simulink model "VSI_GT_avg_il_pll_sv"  (R2016a)
settings: Solver=ode23t  StartTime=0.0  StopTime=0.3  MaxStep=10e-6  RelTol=1e-4  AbsTol=1e-5
values from neighbouring files (symbols this model uses):
  Gdel = Gsvm    [ZVSI_il_tf_cal_sim_comp_frd_PLL_equation.m]    (also in ZVSI_il_tf_cal_sim_comp_frd_model_PQC.m; ZVSI_il_tf_cal_sim_comp_frd_model_v1.m; ZVSI_il_tf_pll_for_shuo.m; ZVSI_ol_pll_share.m)
  Id_ref = (P*Vsd_s-Q*Vsq_s)/(Vsd_s^2+Vsq_s^2)    [ZDQ_GT_DC.m]    (also in ZVSI_il_tf_cal_sim_comp_frd_PLL_equation.m = -10.04; ZVSI_il_tf_cal_sim_comp_frd_model_PQC.m; ZVSI_il_tf_cal_sim_comp_frd_model_v1.m = 1*Id_ref_a(2); ZVSI_il_tf_pll_for_shuo.m = -11.03)
  Iq_ref = (P*Vsq_s+Q*Vsd_s)/(Vsd_s^2+Vsq_s^2)    [ZDQ_GT_DC.m]    (also in ZVSI_il_tf_cal_sim_comp_frd_PLL_equation.m = 0; ZVSI_il_tf_cal_sim_comp_frd_model_PQC.m; ZVSI_il_tf_cal_sim_comp_frd_model_v1.m = 1*Iq_ref_a(2); ZVSI_il_tf_pll_for_shuo.m = 0)
  Ki = tf_filter_dq    [ZVSI_il_tf_cal_sim_comp_frd_PLL_equation.m]    (also in ZVSI_il_tf_cal_sim_comp_frd_model_PQC.m; ZVSI_il_tf_cal_sim_comp_frd_model_v1.m; ZVSI_il_tf_pll_for_shuo.m; ZVSI_ol_pll_zero_pole.m)
  kii = 2*pi*fi*RLboost_con/Vdcref    (= 5.11963247252)    [ZVSI_il_tf_cal_sim_comp_frd_PLL_equation.m]    (also in ZVSI_il_tf_cal_sim_comp_frd_model_PQC.m = ki_i(2)*2*pi*fi*RLboost_con/Vdcref; ZVSI_il_tf_cal_sim_comp_frd_model_v1.m = ki_i(2)*2*pi*fi*RLboost_con/Vdcref; ZVSI_il_tf_pll_for_shuo.m = 25.5982)
  kpi = 2*pi*fi*Lboost_con/Vdcref    (= 0.0465421133865)    [ZVSI_il_tf_cal_sim_comp_frd_PLL_equation.m]    (also in ZVSI_il_tf_cal_sim_comp_frd_model_PQC.m = 0.0232710566933; ZVSI_il_tf_cal_sim_comp_frd_model_v1.m = 0.0232710566933; ZVSI_il_tf_pll_for_shuo.m = 0.0233)
  Kv = tf_filter_dq    [ZVSI_il_tf_cal_sim_comp_frd_PLL_equation.m]    (also in ZVSI_il_tf_cal_sim_comp_frd_model_PQC.m; ZVSI_il_tf_cal_sim_comp_frd_model_v1.m; ZVSI_il_tf_pll_for_shuo.m; ZVSI_ol_pll_zero_pole.m)
  L = 1000e-6    (= 0.001)    [LC_parallel.m]    (also in ZVSI_il_tf_cal_sim_comp_frd_PLL_equation.m; ZVSI_il_tf_cal_sim_comp_frd_model_PQC.m = 0.00097; ZVSI_il_tf_cal_sim_comp_frd_model_v1.m; ZVSI_il_tf_pll_for_shuo.m)
  Lboost_con = 1000e-6    (= 0.001)    [ZVSI_il_tf_cal_sim_comp_frd_PLL_equation.m]    (also in ZVSI_il_tf_cal_sim_comp_frd_model_PQC.m; ZVSI_il_tf_cal_sim_comp_frd_model_v1.m; ZVSI_il_tf_pll_for_shuo.m)
  omega = 2*pi*f    (= 376.991118431)    [ZVSI_il_tf_cal_sim_comp_frd_PLL_equation.m]    (also in ZVSI_il_tf_cal_sim_comp_frd_model_PQC.m = 2513.27412287; ZVSI_il_tf_cal_sim_comp_frd_model_v1.m = 2513.27412287; ZVSI_il_tf_pll_for_shuo.m = 2513.27412287; ZVSI_ol_pll_share.m = 2513.27412287)
  RL = 110e-3    (= 0.11)    [ZVSI_il_tf_cal_sim_comp_frd_PLL_equation.m]    (also in ZVSI_il_tf_cal_sim_comp_frd_model_PQC.m = 0.12; ZVSI_il_tf_cal_sim_comp_frd_model_v1.m; ZVSI_il_tf_pll_for_shuo.m; ZVSI_ol_pll_share.m)
  Vdcref = 270    [ZVSI_il_tf_cal_sim_comp_frd_PLL_equation.m]    (also in ZVSI_il_tf_cal_sim_comp_frd_model_PQC.m; ZVSI_il_tf_cal_sim_comp_frd_model_v1.m; ZVSI_il_tf_pll_for_shuo.m; ZVSI_ol_pll_share.m)
  Vsd_s = Vsdq(1)    [ZDQ_GT_DC.m]    (also in ZVSI_il_tf_cal_sim_comp_frd_PLL_equation.m; ZVSI_il_tf_cal_sim_comp_frd_model_PQC.m; ZVSI_il_tf_cal_sim_comp_frd_model_v1.m; ZVSI_il_tf_pll_for_shuo.m)
libraries: powerlib x23, cstblocks x13, simulink x3
settings Model: Creator=marko  LastModifiedBy=mchssbw3
settings SolverCC: ZeroCrossAlgorithm=Adaptive
settings DataIOCC: LimitDataPoints=on  SaveFormat=Array  SignalLoggingSaveFormat=ModelDataLogs
settings OptimizationCC: BlockReduction=off  DefaultParameterBehavior=Inlined  BufferReuse=off  ExpressionDepthLimit=2147483647
settings DebuggingCC: AlgebraicLoopMsg=none  UnderspecifiedInitializationDetection=Classic  MergeDetectMultiDrivingBlocksExec=none  MultiTaskDSMMsg=warning  MultiTaskCondExecSysMsg=none  UnconnectedInputMsg=none  UnconnectedOutputMsg=none  UnconnectedLineMsg=none  StateNameClashWarn=warning
settings HardwareCC: ProdBitPerPointer=32  ProdLargestAtomicFloat=None  ProdIntDivRoundTo=Undefined  ProdEndianess=Unspecified  ProdWordSize=32  ProdHWDeviceType=32-bit Generic
settings ModelReferenceCC: PropagateSignalLabelsOutOfModel=off
settings GRTTargetCC: CombineOutputUpdateFcns=off  GRTInterface=on
settings ConfigComp: CovModelRefEnable=Off

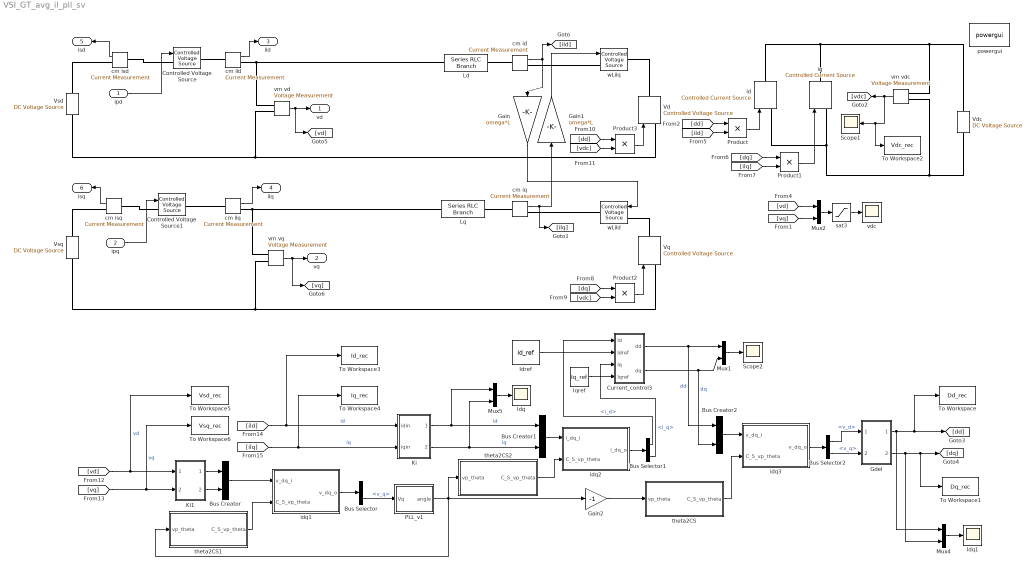
== system VSI_GT_avg_il_pll_sv ==
  ipd : Inport
  ipq : Inport  Port=2
  Bus Creator : BusCreator  Inputs=2
  Bus Creator1 : BusCreator  Inputs=2
  Bus Creator2 : BusCreator  Inputs=2
  Bus Selector : BusSelector  OutputSignals=v_d,v_q
  Bus Selector1 : BusSelector  OutputSignals=i_d,i_q
  Bus Selector2 : BusSelector  OutputSignals=v_d,v_q
  Controlled Voltage Source : powerlib/Electrical Sources/Controlled Voltage Source  Initialize=on  Source_Type=AC  Amplitude=0  Phase=0  Frequency=0  Measurements=None
  Controlled Voltage Source1 : powerlib/Electrical Sources/Controlled Voltage Source  Initialize=on  Source_Type=AC  Amplitude=0  Phase=0  Frequency=0  Measurements=None
  Current_control3 : Subsystem
  Gain : Gain  Gain=omega*L
  Gain1 : Gain  Gain=omega*L
  Gain2 : Gain  Gain=-1
  Gdel : Subsystem
  Idq : Scope
  Idq1 : Scope
  Idref : Constant  Value=Id_ref
  Iqref : Constant  Value=Iq_ref
  Ki : Subsystem
  Ki1 : Subsystem
  Ld : powerlib/Elements/Series RLC Branch  LConnTagsString=__new0  RConnTagsString=__new0  BranchType=RL  Resistance=RL  Inductance=L  SetiL0=off  InitialCurrent=0  Capacitance=1e-6  Setx0=off  InitialVoltage=0  Measurements=None
  Lq : powerlib/Elements/Series RLC Branch  LConnTagsString=__new0  RConnTagsString=__new0  BranchType=RL  Resistance=RL  Inductance=L  SetiL0=off  InitialCurrent=0  Capacitance=1e-6  Setx0=off  InitialVoltage=0  Measurements=None
  Mux{1..2,4..5} (4 alike) : Mux  Inputs=2
  PLL_v1 : Subsystem
  Product{,1..3} (4 alike) : Product  RndMeth=Zero
  Scope1 : Scope
  Scope2 : Scope
  To Workspace : ToWorkspace  VariableName=Dd_rec  SampleTime=-1
  To Workspace1 : ToWorkspace  VariableName=Dq_rec  SampleTime=-1
  To Workspace2 : ToWorkspace  VariableName=Vdc_rec  SampleTime=-1
  To Workspace3 : ToWorkspace  VariableName=Id_rec  SampleTime=-1
  To Workspace4 : ToWorkspace  VariableName=Iq_rec  SampleTime=-1
  To Workspace5 : ToWorkspace  VariableName=Vsd_rec  SampleTime=-1
  To Workspace6 : ToWorkspace  VariableName=Vsq_rec  SampleTime=-1
  Vd : powerlib/Electrical Sources/Controlled Voltage Source  Initialize=on  Source_Type=DC  Amplitude=0  Phase=0  Frequency=0  Measurements=None
  Vdc : powerlib/Electrical Sources/DC Voltage Source  Amplitude=270  Measurements=None
  Vq : powerlib/Electrical Sources/Controlled Voltage Source  Initialize=on  Source_Type=DC  Amplitude=0  Phase=0  Frequency=0  Measurements=None
  Vsd : powerlib/Electrical Sources/DC Voltage Source  Amplitude=Vsd_s  Measurements=None
  Vsq : powerlib/Electrical Sources/DC Voltage Source  Amplitude=0  Measurements=None
  cm id : powerlib/Measurements/Current Measurement  PhasorSimulation=off  OutputType=Complex  PSBequivalent=0
  cm ild : powerlib/Measurements/Current Measurement  PhasorSimulation=off  OutputType=Complex  PSBequivalent=0
  cm ilq : powerlib/Measurements/Current Measurement  PhasorSimulation=off  OutputType=Complex  PSBequivalent=0
  cm iq : powerlib/Measurements/Current Measurement  PhasorSimulation=off  OutputType=Complex  PSBequivalent=0
  cm isd : powerlib/Measurements/Current Measurement  PhasorSimulation=off  OutputType=Complex  PSBequivalent=0
  cm isq : powerlib/Measurements/Current Measurement  PhasorSimulation=off  OutputType=Complex  PSBequivalent=0
  id : powerlib/Electrical Sources/Controlled Current Source  Initialize=on  Source_Type=DC  Amplitude=0  Phase=0  Frequency=0  Measurements=None
  idq1 : Subsystem
  idq2 : Subsystem
  idq3 : Subsystem
  iq : powerlib/Electrical Sources/Controlled Current Source  Initialize=on  Source_Type=DC  Amplitude=0  Phase=0  Frequency=0  Measurements=None
  powergui : powerlib/powergui  Priority=1  SimulationMode=Continuous  SolverType=Tustin  SampleTime=50e-6  frequency=60  SPID=off  DisableSnubberDevices=off  DisableRonSwitches=off  DisableVfSwitches=off  SwTol=0  DisplayEquations=off  Interpol=off  ExternalGateDelay=off  methode=off  Ts=0  FunctionMessages=off  echomessages=off  HookPort=off  EnableUseOfTLC=off  x0status=blocks  frequencyindice=0  Pbase=100e6  ErrMax=1e-4  Iterations=50  UnitsV=kV  UnitsW=MW  buscounter=0  RestoreLinks=warning  ResistiveCurrentMeasurement=off  Frange=[0:2:500]  Ylog=off  Xlog=on  ShowGrid=off  save=off  variable=ZData  structure=0  ZoomFFT=on  StartTime=0.0  cycles=1  DisplayStyle=1  fundamental=60  FreqAxis=off  MaxFrequency=1000  frequencyindicesteady=1  RmsSteady=1  display=off
  sat3 : Saturate  UpperLimit=1000  LowerLimit=0
  theta2CS : Subsystem
  theta2CS1 : Subsystem
  theta2CS2 : Subsystem
  vdc : Scope
  vm vd : powerlib/Measurements/Voltage Measurement  PhasorSimulation=off  OutputType=Complex  PSBequivalent=0
  vm vdc : powerlib/Measurements/Voltage Measurement  PhasorSimulation=off  OutputType=Complex  PSBequivalent=0
  vm vq : powerlib/Measurements/Voltage Measurement  PhasorSimulation=off  OutputType=Complex  PSBequivalent=0
  wLild : powerlib/Electrical Sources/Controlled Voltage Source  Initialize=on  Source_Type=DC  Amplitude=0  Phase=0  Frequency=0  Measurements=None
  wLilq : powerlib/Electrical Sources/Controlled Voltage Source  Initialize=on  Source_Type=DC  Amplitude=0  Phase=0  Frequency=0  Measurements=None
  vd : Outport
  vq : Outport  Port=2
  ild : Outport  Port=3
  ilq : Outport  Port=4
  isd : Outport  Port=5
  isq : Outport  Port=6
  wires:
  cm id/1 -> Gain/1, [ild]
  Gain1/1 -> wLilq/1
  cm iq/1 -> [ilq], Gain1/1
  Gain/1 -> wLild/1
  vm vdc/1 -> [vdc], Scope1/1, To Workspace2/1
  Product/1 -> id/1
  [dd] -> Product/1
  [ild] -> Product/2
  Product1/1 -> iq/1
  [dq] -> Product1/1
  [ilq] -> Product1/2
  [dq] -> Product2/1
  [vdc] -> Product2/2
  Product2/1 -> Vq/1
  [dd] -> Product3/1
  [vdc] -> Product3/2
  Product3/1 -> Vd/1
  vm vd/1 -> vd/1, [vd]
  vm vq/1 -> vq/1, [vq]
  cm ild/1 -> ild/1
  cm ilq/1 -> ilq/1
  cm isd/1 -> isd/1
  cm isq/1 -> isq/1
  Current_control3/1(dd) -> Mux1/1, Bus Creator2/1  "dd"
  Current_control3/2(dq) -> Mux1/2, Bus Creator2/2  "dq"
  Iqref/1 -> Current_control3/4(Iqref)
  Mux1/1 -> Scope2/1
  Mux2/1 -> sat3/1
  sat3/1 -> vdc/1
  PLL_v1/1(angle) -> Gain2/1, theta2CS2/1(vp_theta), theta2CS1/1(vp_theta)
  Gain2/1 -> theta2CS/1(vp_theta)
  Bus Creator/1 -> idq1/1(v_dq_i)
  theta2CS1/1(C_S_vp_theta) -> idq1/2(C_S_vp_theta)
  idq1/1(v_dq_o) -> Bus Selector/1
  Bus Creator1/1 -> idq2/1(i_dq_i)
  idq2/1(i_dq_o) -> Bus Selector1/1
  Bus Selector1/1 -> Current_control3/1(Id)  "<i_d>"
  Bus Selector1/2 -> Current_control3/3(Iq)  "<i_q>"
  theta2CS/1(C_S_vp_theta) -> idq3/2(C_S_vp_theta)
  idq3/1(v_dq_o) -> Bus Selector2/1
  Bus Creator2/1 -> idq3/1(v_dq_i)
  Bus Selector/2 -> PLL_v1/1(Vq)  "<v_q>"
  [vd] -> Mux2/1
  Idref/1 -> Current_control3/2(Idref)
  [ild] -> To Workspace3/1, Ki/1(idin)  "id"
  [ilq] -> To Workspace4/1, Ki/2(iqin)  "iq"
  Mux5/1 -> Idq/1
  Bus Selector2/1 -> Gdel/1(ddin)  "<v_d>"
  Bus Selector2/2 -> Gdel/2(dqin)  "<v_q>"
  Mux4/1 -> Idq1/1
  [vd] -> To Workspace5/1, Ki1/1(idin)  "vd"
  [vq] -> To Workspace6/1, Ki1/2(iqin)  "vq"
  [vq] -> Mux2/2
  theta2CS2/1(C_S_vp_theta) -> idq2/2(C_S_vp_theta)
  Ki1/2(iqout) -> Bus Creator/2
  Ki1/1(idout) -> Bus Creator/1
  Ki/2(iqout) -> Bus Creator1/2, Mux5/2  "iq"
  Ki/1(idout) -> Bus Creator1/1, Mux5/1  "id"
  Gdel/2(dqout) -> [dq], To Workspace1/1, Mux4/2
  Gdel/1(ddout) -> [dd], To Workspace/1, Mux4/1
  ipq/1 -> Controlled Voltage Source1/1
  ipd/1 -> Controlled Voltage Source/1
  connections:
  wLilq/RConn1 -- Vd/RConn1
  wLild/LConn1 -- Vq/RConn1
  cm id/RConn1 -- wLilq/LConn1
  cm id/LConn1 -- Ld/RConn1
  Lq/RConn1 -- cm iq/LConn1
  cm iq/RConn1 -- wLild/RConn1
  Vsd/LConn1 -- Vd/LConn1 -- vm vd/LConn2
  Vq/LConn1 -- vm vq/LConn2 -- Vsq/LConn1
  cm ild/RConn1 -- Ld/LConn1 -- vm vd/LConn1
  cm ilq/RConn1 -- Lq/LConn1 -- vm vq/LConn1
  Vdc/LConn1 -- id/LConn1 -- iq/LConn1 -- vm vdc/LConn2
  cm isd/RConn1 -- Vsd/RConn1
  cm isq/RConn1 -- Vsq/RConn1
  Vdc/RConn1 -- vm vdc/LConn1 -- id/RConn1 -- iq/RConn1
  Controlled Voltage Source/RConn1 -- cm ild/LConn1
  Controlled Voltage Source/LConn1 -- cm isd/LConn1
  Controlled Voltage Source1/RConn1 -- cm ilq/LConn1
  Controlled Voltage Source1/LConn1 -- cm isq/LConn1

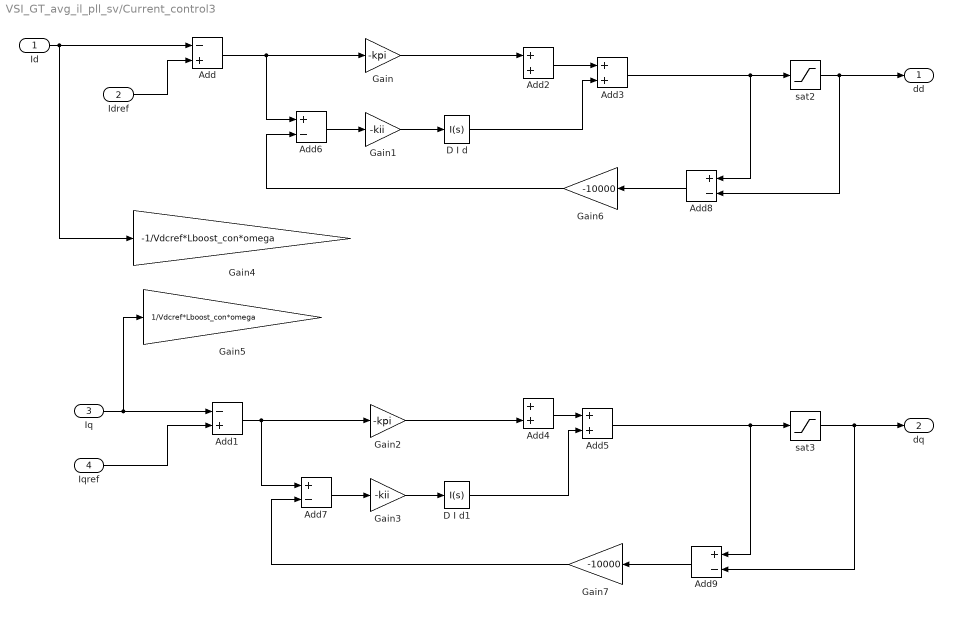
== system VSI_GT_avg_il_pll_sv/Current_control3 ==
  Id : Inport
  Idref : Inport  Port=2
  Iq : Inport  Port=3
  Iqref : Inport  Port=4
  Add : Sum  Inputs=-+
  Add1 : Sum  Inputs=-+
  Add{2..5} (4 alike) : Sum
  Add{6..9} (4 alike) : Sum  Inputs=+-
  D I d : simulink/Continuous/PID Controller  Controller=I  TimeDomain=Continuous-time  SampleTime=-1  IntegratorMethod=Forward Euler  FilterMethod=Forward Euler  Form=Ideal  UseFilter=on  ControllerParametersSource=internal  P=1  I=1  D=0  N=100  InitialConditionSource=internal  InitialConditionForIntegrator=0  InitialConditionForFilter=0  ExternalReset=none  LimitOutput=off  UpperSaturationLimit=inf  LowerSaturationLimit=-inf  LinearizeAsGain=off  AntiWindupMode=none  Kb=1  TrackingMode=off  Kt=1  PParamMin=[]  PParamMax=[]  IParamMin=[]  IParamMax=[]  DParamMin=[]  DParamMax=[]  NParamMin=[]  NParamMax=[]  KbParamMin=[]  KbParamMax=[]  KtParamMin=[]  KtParamMax=[]  POutMin=[]  POutMax=[]  IOutMin=[]  IOutMax=[]  DOutMin=[]  DOutMax=[]  NOutMin=[]  NOutMax=[]  KbOutMin=[]  KbOutMax=[]  KtOutMin=[]  KtOutMax=[]  IntegratorOutMin=[]  IntegratorOutMax=[]  FilterOutMin=[]  FilterOutMax=[]  SumOutMin=[]  SumOutMax=[]  SumI1OutMin=[]  SumI1OutMax=[]  SumI2OutMin=[]  SumI2OutMax=[]  SumI3OutMin=[]  SumI3OutMax=[]  SumDOutMin=[]  SumDOutMax=[]  SaturationOutMin=[]  SaturationOutMax=[]  IntegratorContinuousStateAttributes=''  IntegratorStateMustResolveToSignalObject=off  IntegratorRTWStateStorageClass=Auto  FilterContinuousStateAttributes=''  FilterStateMustResolveToSignalObject=off  FilterRTWStateStorageClass=Auto  DifferentiatorICPrevScaledInput=0  DifferentiatorOutMin=[]  DifferentiatorOutMax=[]
  D I d1 : simulink/Continuous/PID Controller  Controller=I  TimeDomain=Continuous-time  SampleTime=-1  IntegratorMethod=Forward Euler  FilterMethod=Forward Euler  Form=Ideal  UseFilter=on  ControllerParametersSource=internal  P=1  I=1  D=0  N=100  InitialConditionSource=internal  InitialConditionForIntegrator=0  InitialConditionForFilter=0  ExternalReset=none  LimitOutput=off  UpperSaturationLimit=inf  LowerSaturationLimit=-inf  LinearizeAsGain=off  AntiWindupMode=none  Kb=1  TrackingMode=off  Kt=1  PParamMin=[]  PParamMax=[]  IParamMin=[]  IParamMax=[]  DParamMin=[]  DParamMax=[]  NParamMin=[]  NParamMax=[]  KbParamMin=[]  KbParamMax=[]  KtParamMin=[]  KtParamMax=[]  POutMin=[]  POutMax=[]  IOutMin=[]  IOutMax=[]  DOutMin=[]  DOutMax=[]  NOutMin=[]  NOutMax=[]  KbOutMin=[]  KbOutMax=[]  KtOutMin=[]  KtOutMax=[]  IntegratorOutMin=[]  IntegratorOutMax=[]  FilterOutMin=[]  FilterOutMax=[]  SumOutMin=[]  SumOutMax=[]  SumI1OutMin=[]  SumI1OutMax=[]  SumI2OutMin=[]  SumI2OutMax=[]  SumI3OutMin=[]  SumI3OutMax=[]  SumDOutMin=[]  SumDOutMax=[]  SaturationOutMin=[]  SaturationOutMax=[]  IntegratorContinuousStateAttributes=''  IntegratorStateMustResolveToSignalObject=off  IntegratorRTWStateStorageClass=Auto  FilterContinuousStateAttributes=''  FilterStateMustResolveToSignalObject=off  FilterRTWStateStorageClass=Auto  DifferentiatorICPrevScaledInput=0  DifferentiatorOutMin=[]  DifferentiatorOutMax=[]
  Gain : Gain  Gain=-kpi
  Gain1 : Gain  Gain=-kii
  Gain2 : Gain  Gain=-kpi
  Gain3 : Gain  Gain=-kii
  Gain4 : Gain  Gain=-1/Vdcref*Lboost_con*omega
  Gain5 : Gain  Gain=1/Vdcref*Lboost_con*omega
  Gain6 : Gain  Gain=-10000
  Gain7 : Gain  Gain=-10000
  sat2 : Saturate  UpperLimit=1  LowerLimit=-1
  sat3 : Saturate  UpperLimit=1  LowerLimit=-1
  dd : Outport
  dq : Outport  Port=2
  wires:
  Gain7/1 -> Add7/2
  Gain6/1 -> Add6/2
  Add9/1 -> Gain7/1
  Add8/1 -> Gain6/1
  Add3/1 -> sat2/1, Add8/1
  Add7/1 -> Gain3/1
  Add6/1 -> Gain1/1
  sat3/1 -> dq/1, Add9/2
  Add5/1 -> Add9/1, sat3/1
  sat2/1 -> dd/1, Add8/2
  D I d1/1 -> Add5/2
  Add4/1 -> Add5/1
  Gain2/1 -> Add4/2
  Gain3/1 -> D I d1/1
  Add1/1 -> Add7/1, Gain2/1
  Gain/1 -> Add2/1
  D I d/1 -> Add3/2
  Add2/1 -> Add3/1
  Gain1/1 -> D I d/1
  Add/1 -> Add6/1, Gain/1
  Iqref/1 -> Add1/2
  Iq/1 -> Add1/1, Gain5/1
  Idref/1 -> Add/2
  Id/1 -> Gain4/1, Add/1

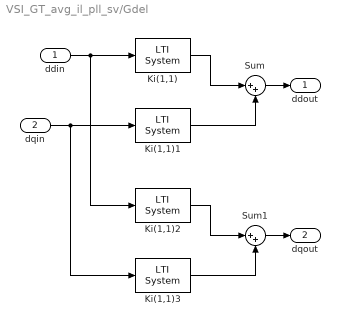
== system VSI_GT_avg_il_pll_sv/Gdel ==
  ddin : Inport
  dqin : Inport  Port=2
  Ki(1,1) : cstblocks/LTI System  sys=Gdel(1,1)  IC=[]
  Ki(1,1)1 : cstblocks/LTI System  sys=Gdel(1,2)  IC=[]
  Ki(1,1)2 : cstblocks/LTI System  sys=Gdel(2,1)  IC=[]
  Ki(1,1)3 : cstblocks/LTI System  sys=Gdel(2,2)  IC=[]
  Sum : Sum  Inputs=|++
  Sum1 : Sum  Inputs=|++
  ddout : Outport
  dqout : Outport  Port=2
  wires:
  Ki(1,1)/1 -> Sum/1
  Ki(1,1)1/1 -> Sum/2
  Ki(1,1)2/1 -> Sum1/1
  Ki(1,1)3/1 -> Sum1/2
  ddin/1 -> Ki(1,1)/1, Ki(1,1)2/1
  dqin/1 -> Ki(1,1)1/1, Ki(1,1)3/1
  Sum/1 -> ddout/1
  Sum1/1 -> dqout/1

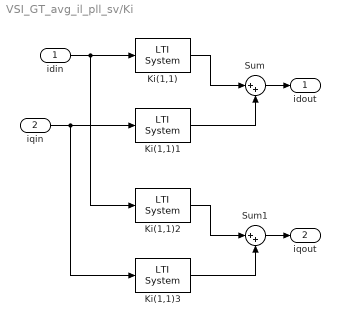
== system VSI_GT_avg_il_pll_sv/Ki ==
  idin : Inport
  iqin : Inport  Port=2
  Ki(1,1) : cstblocks/LTI System  sys=Ki(1,1)  IC=[]
  Ki(1,1)1 : cstblocks/LTI System  sys=Ki(1,2)  IC=[]
  Ki(1,1)2 : cstblocks/LTI System  sys=Ki(2,1)  IC=[]
  Ki(1,1)3 : cstblocks/LTI System  sys=Ki(2,2)  IC=[]
  Sum : Sum  Inputs=|++
  Sum1 : Sum  Inputs=|++
  idout : Outport
  iqout : Outport  Port=2
  wires:
  Ki(1,1)/1 -> Sum/1
  Ki(1,1)1/1 -> Sum/2
  Ki(1,1)2/1 -> Sum1/1
  Ki(1,1)3/1 -> Sum1/2
  idin/1 -> Ki(1,1)/1, Ki(1,1)2/1
  iqin/1 -> Ki(1,1)1/1, Ki(1,1)3/1
  Sum/1 -> idout/1
  Sum1/1 -> iqout/1

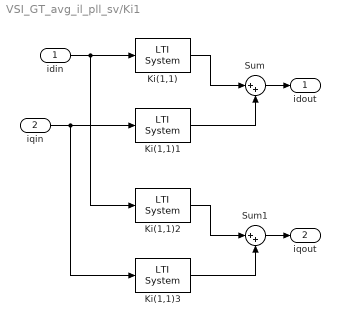
== system VSI_GT_avg_il_pll_sv/Ki1 ==
  idin : Inport
  iqin : Inport  Port=2
  Ki(1,1) : cstblocks/LTI System  sys=Kv(1,1)  IC=[]
  Ki(1,1)1 : cstblocks/LTI System  sys=Kv(1,2)  IC=[]
  Ki(1,1)2 : cstblocks/LTI System  sys=Kv(2,1)  IC=[]
  Ki(1,1)3 : cstblocks/LTI System  sys=Kv(2,2)  IC=[]
  Sum : Sum  Inputs=|++
  Sum1 : Sum  Inputs=|++
  idout : Outport
  iqout : Outport  Port=2
  wires:
  Sum1/1 -> iqout/1
  Sum/1 -> idout/1
  iqin/1 -> Ki(1,1)3/1, Ki(1,1)1/1
  idin/1 -> Ki(1,1)2/1, Ki(1,1)/1
  Ki(1,1)3/1 -> Sum1/2
  Ki(1,1)2/1 -> Sum1/1
  Ki(1,1)1/1 -> Sum/2
  Ki(1,1)/1 -> Sum/1

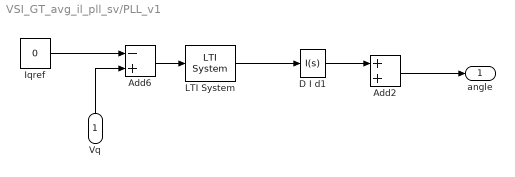
== system VSI_GT_avg_il_pll_sv/PLL_v1 ==
  Vq : Inport
  Add2 : Sum
  Add6 : Sum  Inputs=-+
  D I d1 : simulink/Continuous/PID Controller  Controller=I  TimeDomain=Continuous-time  SampleTime=-1  IntegratorMethod=Forward Euler  FilterMethod=Forward Euler  Form=Ideal  UseFilter=on  ControllerParametersSource=internal  P=1  I=1  D=0  N=100  InitialConditionSource=internal  InitialConditionForIntegrator=0  InitialConditionForFilter=0  ExternalReset=none  LimitOutput=off  UpperSaturationLimit=inf  LowerSaturationLimit=-inf  LinearizeAsGain=off  AntiWindupMode=none  Kb=1  TrackingMode=off  Kt=1  PParamMin=[]  PParamMax=[]  IParamMin=[]  IParamMax=[]  DParamMin=[]  DParamMax=[]  NParamMin=[]  NParamMax=[]  KbParamMin=[]  KbParamMax=[]  KtParamMin=[]  KtParamMax=[]  POutMin=[]  POutMax=[]  IOutMin=[]  IOutMax=[]  DOutMin=[]  DOutMax=[]  NOutMin=[]  NOutMax=[]  KbOutMin=[]  KbOutMax=[]  KtOutMin=[]  KtOutMax=[]  IntegratorOutMin=[]  IntegratorOutMax=[]  FilterOutMin=[]  FilterOutMax=[]  SumOutMin=[]  SumOutMax=[]  SumI1OutMin=[]  SumI1OutMax=[]  SumI2OutMin=[]  SumI2OutMax=[]  SumI3OutMin=[]  SumI3OutMax=[]  SumDOutMin=[]  SumDOutMax=[]  SaturationOutMin=[]  SaturationOutMax=[]  IntegratorContinuousStateAttributes=''  IntegratorStateMustResolveToSignalObject=off  IntegratorRTWStateStorageClass=Auto  FilterContinuousStateAttributes=''  FilterStateMustResolveToSignalObject=off  FilterRTWStateStorageClass=Auto  DifferentiatorICPrevScaledInput=0  DifferentiatorOutMin=[]  DifferentiatorOutMax=[]
  Iqref : Constant  Value=0
  LTI System : cstblocks/LTI System  sys=tf_pll  IC=[]
  angle : Outport
  wires:
  Vq/1 -> Add6/2
  Iqref/1 -> Add6/1
  Add6/1 -> LTI System/1
  LTI System/1 -> D I d1/1
  D I d1/1 -> Add2/1
  Add2/1 -> angle/1

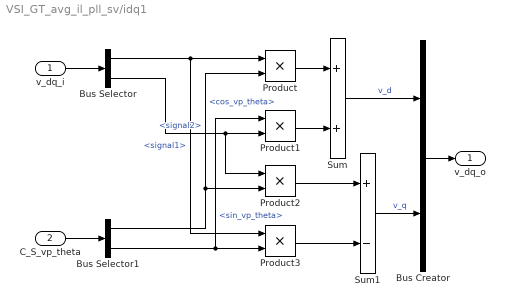
== system VSI_GT_avg_il_pll_sv/idq1 ==
  v_dq_i : Inport
  C_S_vp_theta : Inport  Port=2
  Bus Creator : BusCreator  Inputs=2
  Bus Selector : BusSelector  OutputSignals=signal1,signal2
  Bus Selector1 : BusSelector  OutputSignals=cos_vp_theta,sin_vp_theta
  Product{,1..3} (4 alike) : Product  RndMeth=Zero
  Sum : Sum
  Sum1 : Sum  Inputs=+-
  v_dq_o : Outport
  wires:
  Bus Creator/1 -> v_dq_o/1
  v_dq_i/1 -> Bus Selector/1
  Bus Selector/1 -> Product/1, Product3/1  "<signal1>"
  Bus Selector/2 -> Product1/2, Product2/1  "<signal2>"
  C_S_vp_theta/1 -> Bus Selector1/1
  Bus Selector1/1 -> Product/2, Product2/2  "<cos_vp_theta>"
  Bus Selector1/2 -> Product1/1, Product3/2  "<sin_vp_theta>"
  Product/1 -> Sum/1
  Product1/1 -> Sum/2
  Product2/1 -> Sum1/1
  Product3/1 -> Sum1/2
  Sum/1 -> Bus Creator/1  "v_d"
  Sum1/1 -> Bus Creator/2  "v_q"

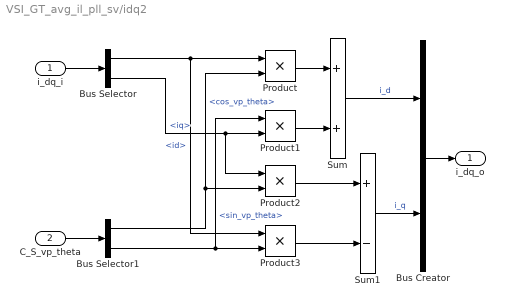
== system VSI_GT_avg_il_pll_sv/idq2 ==
  i_dq_i : Inport
  C_S_vp_theta : Inport  Port=2
  Bus Creator : BusCreator  Inputs=2
  Bus Selector : BusSelector  OutputSignals=id,iq
  Bus Selector1 : BusSelector  OutputSignals=cos_vp_theta,sin_vp_theta
  Product{,1..3} (4 alike) : Product  RndMeth=Zero
  Sum : Sum
  Sum1 : Sum  Inputs=+-
  i_dq_o : Outport
  wires:
  Bus Creator/1 -> i_dq_o/1
  i_dq_i/1 -> Bus Selector/1
  Bus Selector/1 -> Product/1, Product3/1  "<id>"
  Bus Selector/2 -> Product1/2, Product2/1  "<iq>"
  C_S_vp_theta/1 -> Bus Selector1/1
  Bus Selector1/1 -> Product/2, Product2/2  "<cos_vp_theta>"
  Bus Selector1/2 -> Product1/1, Product3/2  "<sin_vp_theta>"
  Product/1 -> Sum/1
  Product1/1 -> Sum/2
  Product2/1 -> Sum1/1
  Product3/1 -> Sum1/2
  Sum/1 -> Bus Creator/1  "i_d"
  Sum1/1 -> Bus Creator/2  "i_q"

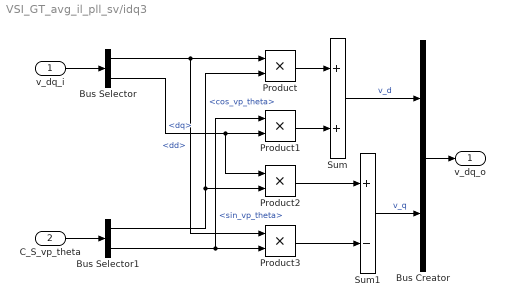
== system VSI_GT_avg_il_pll_sv/idq3 ==
  v_dq_i : Inport
  C_S_vp_theta : Inport  Port=2
  Bus Creator : BusCreator  Inputs=2
  Bus Selector : BusSelector  OutputSignals=dd,dq
  Bus Selector1 : BusSelector  OutputSignals=cos_vp_theta,sin_vp_theta
  Product{,1..3} (4 alike) : Product  RndMeth=Zero
  Sum : Sum
  Sum1 : Sum  Inputs=+-
  v_dq_o : Outport
  wires:
  Sum1/1 -> Bus Creator/2  "v_q"
  Sum/1 -> Bus Creator/1  "v_d"
  Product3/1 -> Sum1/2
  Product2/1 -> Sum1/1
  Product1/1 -> Sum/2
  Product/1 -> Sum/1
  Bus Selector1/2 -> Product3/2, Product1/1  "<sin_vp_theta>"
  Bus Selector1/1 -> Product2/2, Product/2  "<cos_vp_theta>"
  C_S_vp_theta/1 -> Bus Selector1/1
  Bus Selector/2 -> Product2/1, Product1/2  "<dq>"
  Bus Selector/1 -> Product3/1, Product/1  "<dd>"
  v_dq_i/1 -> Bus Selector/1
  Bus Creator/1 -> v_dq_o/1

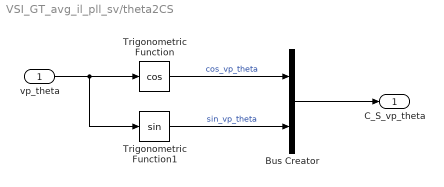
== system VSI_GT_avg_il_pll_sv/theta2CS ==
  vp_theta : Inport
  Bus Creator : BusCreator  Inputs=2
  Trigonometric Function : Trigonometry  Operator=cos  OutputSignalType=real
  Trigonometric Function1 : Trigonometry  OutputSignalType=real
  C_S_vp_theta : Outport
  wires:
  Bus Creator/1 -> C_S_vp_theta/1
  vp_theta/1 -> Trigonometric Function/1, Trigonometric Function1/1
  Trigonometric Function/1 -> Bus Creator/1  "cos_vp_theta"
  Trigonometric Function1/1 -> Bus Creator/2  "sin_vp_theta"

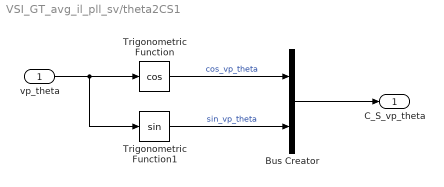
== system VSI_GT_avg_il_pll_sv/theta2CS1 ==
  vp_theta : Inport
  Bus Creator : BusCreator  Inputs=2
  Trigonometric Function : Trigonometry  Operator=cos
  Trigonometric Function1 : Trigonometry
  C_S_vp_theta : Outport
  wires:
  Trigonometric Function1/1 -> Bus Creator/2  "sin_vp_theta"
  Trigonometric Function/1 -> Bus Creator/1  "cos_vp_theta"
  vp_theta/1 -> Trigonometric Function1/1, Trigonometric Function/1
  Bus Creator/1 -> C_S_vp_theta/1

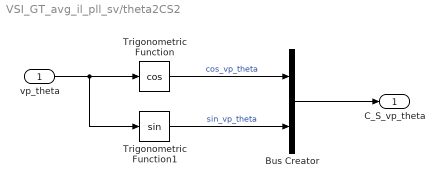
== system VSI_GT_avg_il_pll_sv/theta2CS2 ==
  vp_theta : Inport
  Bus Creator : BusCreator  Inputs=2
  Trigonometric Function : Trigonometry  Operator=cos
  Trigonometric Function1 : Trigonometry
  C_S_vp_theta : Outport
  wires:
  Bus Creator/1 -> C_S_vp_theta/1
  vp_theta/1 -> Trigonometric Function/1, Trigonometric Function1/1
  Trigonometric Function/1 -> Bus Creator/1  "cos_vp_theta"
  Trigonometric Function1/1 -> Bus Creator/2  "sin_vp_theta"
